simulink model "integr_servicing"  (R2024a)
settings: Solver=VariableStepAuto  StartTime=0.0  StopTime=10.0  RelTol=1e-3
settings Model: Creator=r.de-oliveira  LastModifiedBy=r.de-oliveira
settings ModelReferenceCC: EnableRefExpFcnMdlSchedulingChecks=on
settings RTWCC: GPUComputeCapability=3.5

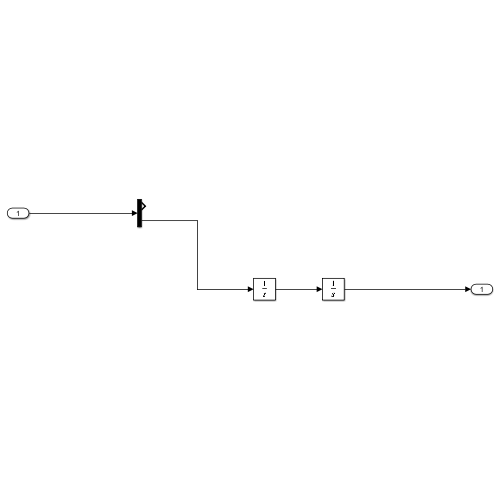
[thumbnail: Simulink's stored preview of the top-level diagram]
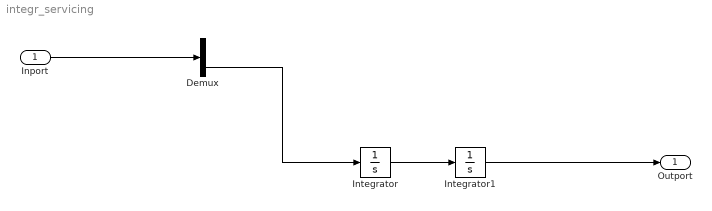
== system integr_servicing ==
  Inport : Inport  PortDimensions=6
  Demux : Demux  Outputs=[3 3]
  Integrator : Integrator
  Integrator1 : Integrator
  Outport : Outport  PortDimensions=3
  wires:
  Integrator1/1 -> Outport/1
  Integrator/1 -> Integrator1/1
  Inport/1 -> Demux/1
  Demux/2 -> Integrator/1
